simulink model "SF014A_InertiaCmpVel"  (R2013b)
settings: Solver=FixedStepDiscrete  SolverMode=SingleTasking  StartTime=0.0  StopTime=10  FixedStep=0.002  RelTol=1e-3
undefined symbols (not defined in the file): ARCHGLBPRM_2MILLISEC_SEC_F32, ARCHGLBPRM_2PI_ULS_F32, ARCHGLBPRM_PIOVER180_ULS_F32, FLTINJ_INERTIACMPVEL_INERTIACMPCMD, InertiaCmpVelDampgDecelGain, InertiaCmpVelDampgDecelGainFallSlew, InertiaCmpVelDampgGainOffThd, InertiaCmpVelDampgGainOnThd, InertiaCmpVelDecelGainEnaCal, InertiaCmpVelMotInertia, InertiaCmpVelNotchFilStruct, NOTCHFILZEROTHD_ULS_F32, SysGlbPrmSysKineRat, SysGlbPrmTorsBarStfn
libraries: FixdToFloat x13, LnrIntrpn x13, FloatToFixd x9, NxtrAbslt x4, NxtrMath x4, NxtrLim x4, simulink x2, Fil x2
(part 1 of 3)
Description:
  | Provide compensation that is dependent on filtering of motor velocity.  Primary purpose is to compensate for motor inertia
  | at low frequencies and provide damping acting at higher frequencies.
  | 
  | This function requires SF-00 Common Calibrations.
settings Model: Creator=xzqqlw  LastModifiedBy=XZB1DB
settings SolverCC: AutoInsertRateTranBlk=on  InsertRTBMode=Always
settings DataIOCC: LimitDataPoints=off  SaveFormat=Structure  ReturnWorkspaceOutputs=on
settings OptimizationCC: BlockReduction=off  InlineParams=on  ZeroExternalMemoryAtStartup=off  ZeroInternalMemoryAtStartup=off  OptimizeModelRefInitCode=on  LifeSpan=1
settings DebuggingCC: SignalInfNanChecking=error  SignalRangeChecking=warning  UnderspecifiedInitializationDetection=Simplified  SolverPrmCheckMsg=error  InheritedTsInSrcMsg=error  DiscreteInheritContinuousMsg=error  SingleTaskRateTransMsg=error  TasksWithSamePriorityMsg=error  SigSpecEnsureSampleTimeMsg=error  CheckMatrixSingularityMsg=error  ParameterUnderflowMsg=error  ParameterPrecisionLossMsg=error  ParameterTunabilityLossMsg=error  FixptConstUnderflowMsg=warning  FixptConstOverflowMsg=warning  VectorMatrixConversionMsg=error  SignalLabelMismatchMsg=error  UnconnectedInputMsg=error  UnconnectedOutputMsg=error  UnconnectedLineMsg=error  SFcnCompatibilityMsg=error  UniqueDataStoreMsg=warning  BusObjectLabelMismatch=error  RootOutportRequireBusObject=error  AssertControl=DisableAll  ModelReferenceIOMsg=error  ModelReferenceVersionMismatchMessage=warning  ModelReferenceIOMismatchMessage=error  ModelReferenceCSMismatchMessage=warning  ModelReferenceDataLoggingMessage=error  StateNameClashWarn=warning  StrictBusMsg=ErrorOnBusTreatedAsVector  NonBusSignalsTreatedAsBus=error  SFUnexpectedBacktrackingDiag=error  SFInvalidInputDataAccessInChartInitDiag=error  SFNoUnconditionalDefaultTransitionDiag=error  SFTransitionOutsideNaturalParentDiag=error  SFUnconditionalTransitionShadowingDiag=error  SFUndirectedBroadcastEventsDiag=error
settings ModelReferenceCC: ModelReferenceNumInstancesAllowed=Single
settings RTWCC: SystemTargetFile=autosar.tlc  GenCodeOnly=on  TemplateMakefile=ert_default_tmf  Description=AUTOSAR  GenerateReport=on  ProcessScript=autosar_make_rtw_hook  LaunchReport=on
settings CodeAppCC: GenerateComments=off  IgnoreCustomStorageClasses=off  CustomSymbolStrType=$N$R$M  CustomSymbolStrBlkIO=$N$M  SimulinkBlockComments=off
settings STFCustomTargetCC: ParMdlRefBuildCompliant=on  CompOptLevelCompliant=on  IncludeMdlTerminateFcn=off  CombineOutputUpdateFcns=on  SuppressErrorStatus=on  ERTFirstTimeCompliant=on  ERTCustomFileBanners=on  SupportNonFinite=off  SupportComplex=off  SupportContinuousTime=off  SupportNonInlinedSFcns=off  MATLABClassNameForMDSCustomization=Simulink.SoftwareTarget.ERTCustomization  AutosarCompliant=on  GRTInterface=off  SystemTargetFile=autosar.tlc
settings ERTTargetCC: CodeReplacementLibrary=ANSI_C  ConcurrentExecutionCompliant=off  IncludeMdlTerminateFcn=off  SuppressErrorStatus=on  SupportNonFinite=off  SupportComplex=off  ModelStepFunctionPrototypeControlCompliant=off  CPPClassGenCompliant=off  AutosarCompliant=on  InlinedParameterPlacement=NonHierarchical  ERTCustomFileTemplate=example_file_process.tlc  EnableUserReplacementTypes=on

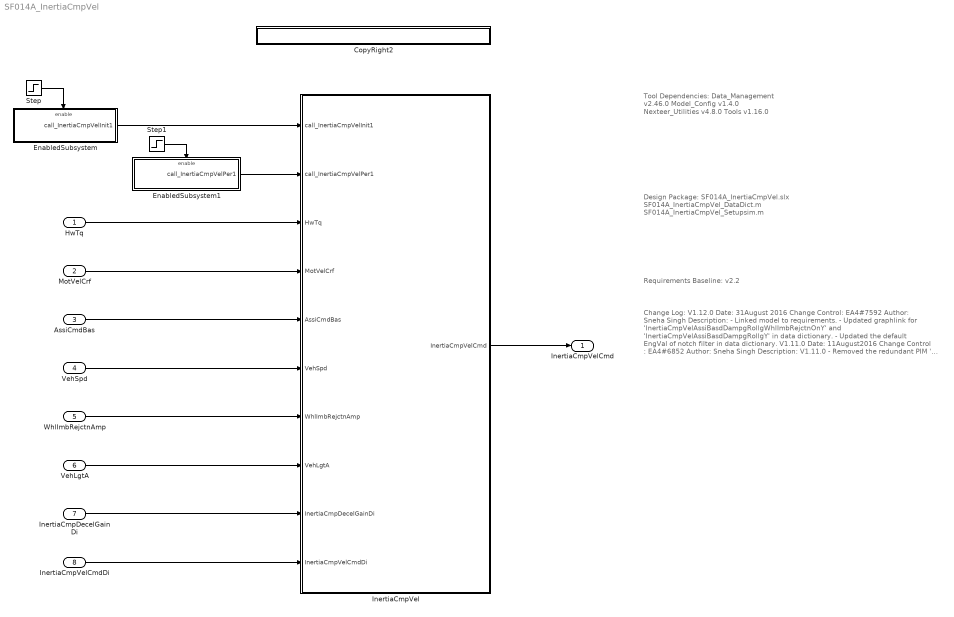
== system SF014A_InertiaCmpVel ==
  note: Requirements Baseline: v2.2
  note: Design Package:
      | SF014A_InertiaCmpVel.slx
      | SF014A_InertiaCmpVel_DataDict.m
      | SF014A_InertiaCmpVel_Setupsim.m
  note: Tool Dependencies:
      |
      | Data_Management v2.46.0
      | Model_Config v1.4.0
      | Nexteer_Utilities v4.8.0
      | Tools v1.16.0
  note: Change Log:
      |
      | V1.12.0
      | Date: 31August 2016
      | Change Control: EA4#7592
      | Author: Sneha Singh
      | Description:
      | - Linked model to requirements.
      | - Updated graphlink for 'InertiaCmpVelAssiBasdDampgRollgWhlImbRejctnOnY' and
      | 'InertiaCmpVelAssiBasdDampgRollgY' in data dictionary.
      | - Updated the default EngVal of notch filter in data dictionary.
      |
      | V1.11.0
      | Date: 11August2016
      | Change Control : EA4#6852
      | Author: Sneha Singh
      |
      | Description:
      | V1.11.0
      | - Removed the redundant PIM ' DecelGainPrev' and the display variable 'dInertiaCmpVelDecelGain '.
      | V1.10.0
      | - Conversion from Level 0 to Level 3 model.
      | - Names of PIM blocks have been updated as per EA4 standards in model and DD.
      | - Range of Filter Gain and State Variable for 'TqSnsrVelFil' updated in the data dictionary.
      | - Added the graphlink property for 'InertiaCmpVelNotchBlndY' in the data dictionary.
      | V1.9.0
      | - Modified datatype of Input 'InertiaCmpDecelGainDi' in the data dictionary.
      | - Added the Cal 'InertiaCmpVelDecelGainEnaCal' to data dictionary and model.
      | V1.8.0
      | - Modified datatype of PIM variable 'NotchFilChk'
      | V1.7.0
      | - Added the PIM variable 'NotchFilChk'
      | - Modified the 'Inertia Comp Notch Compensation' block.
      | - Added a saturation block to the velocity output in the block 'DriverVelCalc'.
      | Added a saturation block to the Inertia Comp output in the block 'GenFddIcCmd'.
      | - Added the input 'InertiaCmpDecelGainDi' to the model.
      | - Changes in the limits of some PIM variables in data dictionary.
      | V1.6.0
      | - Few simulink model properties changed (specifically initial conditions)
      |  so that the simulation can run.
      | - Changes in the limits of some PIM variables in data dictionary.
      | V1.5.0
      | - DriverVelCalc block modified to add motor velocity for the output (Simulink
      | model/design modification)
      | - Changes in the limits of some PIM variables in data dictionary.
      | - The min/max and default value of InertiaCmpVelDampgDecelGainFallSlew
      | V1.4.0
      | - Changes in the limits of some display variables in data dictionary.
      | - Few simulink model properties changes so that the simulation can run.
      | V1.3.0
      | - No changes to model or data dictionary.
      | - Added an init.txt file for initialization
      | were modified in data dictionary.
      | V1.2.0
      | - Minor changes to data dictionary
      |  and default cals.
      | V1.1.0
      | - Minor changes to data dictionary
      | V1.0.0
      | - Initial Release
      | - Based on EA3 version 006
      | - Notch Filter Added
  HwTq : Inport  OutDataTypeStr=single
  MotVelCrf : Inport  Port=2  OutDataTypeStr=single
  AssiCmdBas : Inport  Port=3  OutDataTypeStr=single
  VehSpd : Inport  Port=4  OutDataTypeStr=single
  WhlImbRejctnAmp : Inport  Port=5  OutDataTypeStr=single
  VehLgtA : Inport  Port=6  OutDataTypeStr=single
  InertiaCmpDecelGainDi : Inport  Port=7  OutDataTypeStr=single
  InertiaCmpVelCmdDi : Inport  Port=8  OutDataTypeStr=single
  CopyRight2 : Subsystem  Description=|  mask(Copyright Information){none=on}
      | Copyright info block.                                               
      |                                                                     
      | Place copyright information at the top of every subsystem in design.
      mask prompts: none "No parameters"
      mask help: Place copyright information at the top of every subsystem in design.
      mask Display:
      | NxtrConf = 'Nexteer Confidential';
      | 
      | sys = bdroot; %handle for the current model ("system")
      | first = get_param(sys,'Created');
      | first = first(end-3:end);  %year is last four digits
      | 
      | last = get_param(sys,'LastModifiedDate');
      | if isempty(last)
      |     last = datestr(now,'yyyy');
      | else
      |     last = last(end-3:end);
      | end
      | 
      | if strcmp(first,last)
      |     fprintf('%s -- Copyright %s Nexteer',NxtrConf,first)
      | else
      |     fprintf('%s -- %s%s- %s Nexteer',NxtrConf,char(169),first,last)
      | end
  EnabledSubsystem : Subsystem  TreatAsAtomicUnit=on
  EnabledSubsystem1 : Subsystem  TreatAsAtomicUnit=on
  InertiaCmpVel : Subsystem
  Step : Step  Time=0  Before=1  After=0  SampleTime=0
  Step1 : Step  Time=0  SampleTime=0.002
  InertiaCmpVelCmd : Outport
  wires:
  AssiCmdBas/1 -> InertiaCmpVel/5(AssiCmdBas)
  VehSpd/1 -> InertiaCmpVel/6(VehSpd)
  WhlImbRejctnAmp/1 -> InertiaCmpVel/7(WhlImbRejctnAmp)
  HwTq/1 -> InertiaCmpVel/3(HwTq)
  MotVelCrf/1 -> InertiaCmpVel/4(MotVelCrf)
  InertiaCmpVel/1(InertiaCmpVelCmd) -> InertiaCmpVelCmd/1
  InertiaCmpVelCmdDi/1 -> InertiaCmpVel/10(InertiaCmpVelCmdDi)
  VehLgtA/1 -> InertiaCmpVel/8(VehLgtA)
  Step/1 -> EnabledSubsystem/Enable
  EnabledSubsystem1/1(call_InertiaCmpVelPer1) -> InertiaCmpVel/2(call_InertiaCmpVelPer1)
  EnabledSubsystem/1(call_InertiaCmpVelInit1) -> InertiaCmpVel/1(call_InertiaCmpVelInit1)
  Step1/1 -> EnabledSubsystem1/Enable
  InertiaCmpDecelGainDi/1 -> InertiaCmpVel/9(InertiaCmpDecelGainDi)

== system SF014A_InertiaCmpVel/CopyRight2 ==

== system SF014A_InertiaCmpVel/EnabledSubsystem ==
  Enable : EnablePort
  CopyRight2 : Subsystem  Description=|  mask(Copyright Information){none=on}
      | Copyright info block.                                               
      |                                                                     
      | Place copyright information at the top of every subsystem in design.
      mask prompts: none "No parameters"
      mask help: Place copyright information at the top of every subsystem in design.
      mask Display:
      | NxtrConf = 'Nexteer Confidential';
      | 
      | sys = bdroot; %handle for the current model ("system")
      | first = get_param(sys,'Created');
      | if(isempty(first))
      |     first = datestr(now,'yyyy');
      | else
      |     first = first(end-3:end);  %year is last four digits
      | end
      | 
      | last = get_param(sys,'LastModifiedDate');
      | if isempty(last)
      |     last = datestr(now,'yyyy');
      | else
      |     last = last(end-3:end);
      | end
      | 
      | if strcmp(first,last)
      |     fprintf('%s -- Copyright %s Nexteer',NxtrConf,first)
      | else
      |     fprintf('%s -- %s%s- %s Nexteer',NxtrConf,char(169),first,last)
      | end
  Function-Call Generator1 : simulink/Ports & Subsystems/Function-Call Generator  sample_time=0  numberOfIterations=1
  call_InertiaCmpVelInit1 : Outport
  wires:
  Function-Call Generator1/1 -> call_InertiaCmpVelInit1/1

== system SF014A_InertiaCmpVel/EnabledSubsystem1 ==
  Enable : EnablePort
  CopyRight2 : Subsystem  Description=|  mask(Copyright Information){none=on}
      | Copyright info block.                                               
      |                                                                     
      | Place copyright information at the top of every subsystem in design.
      mask prompts: none "No parameters"
      mask help: Place copyright information at the top of every subsystem in design.
      mask Display:
      | NxtrConf = 'Nexteer Confidential';
      | 
      | sys = bdroot; %handle for the current model ("system")
      | first = get_param(sys,'Created');
      | if(isempty(first))
      |     first = datestr(now,'yyyy');
      | else
      |     first = first(end-3:end);  %year is last four digits
      | end
      | 
      | last = get_param(sys,'LastModifiedDate');
      | if isempty(last)
      |     last = datestr(now,'yyyy');
      | else
      |     last = last(end-3:end);
      | end
      | 
      | if strcmp(first,last)
      |     fprintf('%s -- Copyright %s Nexteer',NxtrConf,first)
      | else
      |     fprintf('%s -- %s%s- %s Nexteer',NxtrConf,char(169),first,last)
      | end
  Function-Call Generator1 : simulink/Ports & Subsystems/Function-Call Generator  sample_time=0.002  numberOfIterations=1
  call_InertiaCmpVelPer1 : Outport
  wires:
  Function-Call Generator1/1 -> call_InertiaCmpVelPer1/1

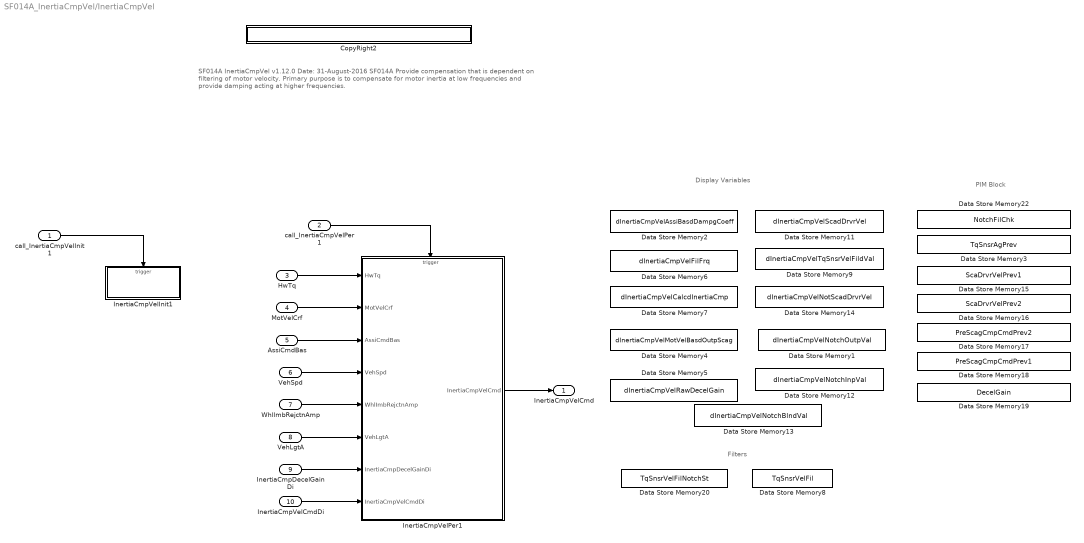
== system SF014A_InertiaCmpVel/InertiaCmpVel ==
  note: Display Variables
  note: SF014A  InertiaCmpVel
      | v1.12.0 														Date: 31-August-2016
      |
      | SF014A
      | Provide compensation that is dependent on filtering
      | of motor velocity. Primary purpose is to compensate for motor inertia at
      | low frequencies and provide damping acting at higher frequencies.
  note: PIM Block
  note: Filters
  call_InertiaCmpVelInit1 : Inport
  call_InertiaCmpVelPer1 : Inport  Port=2
  HwTq : Inport  RequirementInfo="{'linktype_rmi_doors' '0000a52e (/E-STEER Core/SubSystem Specifications/Application Functions/SF014A Inertia Compensation)' '#SF014A_9' 'true' 'REQ:  SF014A_9' '' } %GIDa_f01b9146_b334_492a_9ec3_b1b2beaf36fa"  Port=3  OutDataTypeStr=single
  MotVelCrf : Inport  RequirementInfo="{'linktype_rmi_doors' '0000a52e (/E-STEER Core/SubSystem Specifications/Application Functions/SF014A Inertia Compensation)' '#SF014A_32' 'true' 'REQ:  SF014A_32' '' } %GIDa_a3fb682f_8b72_444f_8c20_ec5397ad6a39"  Port=4  OutDataTypeStr=single
  AssiCmdBas : Inport  RequirementInfo="{'linktype_rmi_doors' '0000a52e (/E-STEER Core/SubSystem Specifications/Application Functions/SF014A Inertia Compensation)' '#SF014A_33' 'true' 'REQ:  SF014A_33' '' } %GIDa_d5627f17_e36b_4ebf_b0c3_bf571987fd69"  Port=5  OutDataTypeStr=single
  VehSpd : Inport  RequirementInfo="{'linktype_rmi_doors' '0000a52e (/E-STEER Core/SubSystem Specifications/Application Functions/SF014A Inertia Compensation)' '#SF014A_34' 'true' 'REQ:  SF014A_34' '' } %GIDa_30fe50f3_e3d5_4c85_a02f_97c34158807d"  Port=6  OutDataTypeStr=single
  WhlImbRejctnAmp : Inport  RequirementInfo="{'linktype_rmi_doors' '0000a52e (/E-STEER Core/SubSystem Specifications/Application Functions/SF014A Inertia Compensation)' '#SF014A_35' 'true' 'REQ:  SF014A_35' '' } %GIDa_6689df3e_a07a_4416_91b0_faa74f28addd"  Port=7  OutDataTypeStr=single
  VehLgtA : Inport  RequirementInfo="{'linktype_rmi_doors' '0000a52e (/E-STEER Core/SubSystem Specifications/Application Functions/SF014A Inertia Compensation)' '#SF014A_37' 'true' 'REQ:  SF014A_37' '' } %GIDa_068774d9_b29a_42bf_9303_5199fc3935e8"  Port=8  OutDataTypeStr=single
  InertiaCmpDecelGainDi : Inport  RequirementInfo="{'linktype_rmi_doors' '0000a52e (/E-STEER Core/SubSystem Specifications/Application Functions/SF014A Inertia Compensation)' '#SF014A_64' 'true' 'REQ:  SF014A_64' '' } %GIDa_847a8fc7_5162_4283_91ca_d0e4dd3290d5"  Port=9  OutDataTypeStr=single
  InertiaCmpVelCmdDi : Inport  RequirementInfo="{'linktype_rmi_doors' '0000a52e (/E-STEER Core/SubSystem Specifications/Application Functions/SF014A Inertia Compensation)' '#SF014A_36' 'true' 'REQ:  SF014A_36' '' } %GIDa_8753a04c_012b_41bc_9ba5_be465b9c35dc"  Port=10  OutDataTypeStr=single
  CopyRight2 : Subsystem  Description=|  mask(Copyright Information){none=on}
      | Copyright info block.                                               
      |                                                                     
      | Place copyright information at the top of every subsystem in design.
      mask prompts: none "No parameters"
      mask help: Place copyright information at the top of every subsystem in design.
      mask Display:
      | NxtrConf = 'Nexteer Confidential';
      | 
      | sys = bdroot; %handle for the current model ("system")
      | first = get_param(sys,'Created');
      | first = first(end-3:end);  %year is last four digits
      | 
      | last = get_param(sys,'LastModifiedDate');
      | if isempty(last)
      |     last = datestr(now,'yyyy');
      | else
      |     last = last(end-3:end);
      | end
      | 
      | if strcmp(first,last)
      |     fprintf('%s -- Copyright %s Nexteer',NxtrConf,first)
      | else
      |     fprintf('%s -- %s%s- %s Nexteer',NxtrConf,char(169),first,last)
      | end
  Data Store Memory1 : DataStoreMemory  DataStoreName=dInertiaCmpVelNotchOutpVal  ReadBeforeWriteMsg=warning  WriteAfterWriteMsg=warning  WriteAfterReadMsg=warning  StateMustResolveToSignalObject=on
  Data Store Memory11 : DataStoreMemory  DataStoreName=dInertiaCmpVelScadDrvrVel  ReadBeforeWriteMsg=warning  WriteAfterWriteMsg=warning  WriteAfterReadMsg=warning  StateMustResolveToSignalObject=on
  Data Store Memory12 : DataStoreMemory  DataStoreName=dInertiaCmpVelNotchInpVal  ReadBeforeWriteMsg=warning  WriteAfterWriteMsg=warning  WriteAfterReadMsg=warning  StateMustResolveToSignalObject=on
  Data Store Memory13 : DataStoreMemory  DataStoreName=dInertiaCmpVelNotchBlndVal  ReadBeforeWriteMsg=warning  WriteAfterWriteMsg=warning  WriteAfterReadMsg=warning  StateMustResolveToSignalObject=on
  Data Store Memory14 : DataStoreMemory  DataStoreName=dInertiaCmpVelNotScadDrvrVel  ReadBeforeWriteMsg=warning  WriteAfterWriteMsg=warning  WriteAfterReadMsg=warning  StateMustResolveToSignalObject=on
  Data Store Memory15 : DataStoreMemory  DataStoreName=ScaDrvrVelPrev1  StateMustResolveToSignalObject=on
  Data Store Memory16 : DataStoreMemory  DataStoreName=ScaDrvrVelPrev2  StateMustResolveToSignalObject=on
  Data Store Memory17 : DataStoreMemory  DataStoreName=PreScagCmpCmdPrev2  StateMustResolveToSignalObject=on
  Data Store Memory18 : DataStoreMemory  DataStoreName=PreScagCmpCmdPrev1  StateMustResolveToSignalObject=on
  Data Store Memory19 : DataStoreMemory  DataStoreName=DecelGain  StateMustResolveToSignalObject=on
  Data Store Memory2 : DataStoreMemory  DataStoreName=dInertiaCmpVelAssiBasdDampgCoeff  ReadBeforeWriteMsg=warning  WriteAfterWriteMsg=warning  WriteAfterReadMsg=warning  StateMustResolveToSignalObject=on
  Data Store Memory20 : DataStoreMemory  DataStoreName=TqSnsrVelFilNotchSt  ReadBeforeWriteMsg=warning  WriteAfterWriteMsg=warning  WriteAfterReadMsg=warning  InitialValue=[]  StateMustResolveToSignalObject=on
  Data Store Memory22 : DataStoreMemory  RequirementInfo="{'linktype_rmi_doors' '0000a52e (/E-STEER Core/SubSystem Specifications/Application Functions/SF014A Inertia Compensation)' '#SF014A_94' 'true' 'REQ:  SF014A_94' '' } %GIDa_2f01161b_bb81_48fb_9c8e_b5cf915a9566"  DataStoreName=NotchFilChk  StateMustResolveToSignalObject=on
  Data Store Memory3 : DataStoreMemory  DataStoreName=TqSnsrAgPrev  StateMustResolveToSignalObject=on
  Data Store Memory4 : DataStoreMemory  DataStoreName=dInertiaCmpVelMotVelBasdOutpScag  ReadBeforeWriteMsg=warning  WriteAfterWriteMsg=warning  WriteAfterReadMsg=warning  StateMustResolveToSignalObject=on
  Data Store Memory5 : DataStoreMemory  DataStoreName=dInertiaCmpVelRawDecelGain  ReadBeforeWriteMsg=warning  WriteAfterWriteMsg=warning  WriteAfterReadMsg=warning  StateMustResolveToSignalObject=on
  Data Store Memory6 : DataStoreMemory  DataStoreName=dInertiaCmpVelFilFrq  ReadBeforeWriteMsg=warning  WriteAfterWriteMsg=warning  WriteAfterReadMsg=warning  StateMustResolveToSignalObject=on
  Data Store Memory7 : DataStoreMemory  DataStoreName=dInertiaCmpVelCalcdInertiaCmp  ReadBeforeWriteMsg=warning  WriteAfterWriteMsg=warning  WriteAfterReadMsg=warning  StateMustResolveToSignalObject=on
  Data Store Memory8 : DataStoreMemory  DataStoreName=TqSnsrVelFil  InitialValue=[]  OutDataTypeStr=Bus: FilLpRec1  StateMustResolveToSignalObject=on
  Data Store Memory9 : DataStoreMemory  DataStoreName=dInertiaCmpVelTqSnsrVelFildVal  ReadBeforeWriteMsg=warning  WriteAfterWriteMsg=warning  WriteAfterReadMsg=warning  StateMustResolveToSignalObject=on
  InertiaCmpVelInit1 : Subsystem  TreatAsAtomicUnit=on
  InertiaCmpVelPer1 : Subsystem
  InertiaCmpVelCmd : Outport  RequirementInfo="{'linktype_rmi_doors' '0000a52e (/E-STEER Core/SubSystem Specifications/Application Functions/SF014A Inertia Compensation)' '#SF014A_11' 'true' 'REQ:  SF014A_11' '' } %GIDa_b766a6be_ddbc_4ccc_baa7_69f83a871e7a"
  wires:
  InertiaCmpVelPer1/1(InertiaCmpVelCmd) -> InertiaCmpVelCmd/1
  AssiCmdBas/1 -> InertiaCmpVelPer1/3(AssiCmdBas)
  VehSpd/1 -> InertiaCmpVelPer1/4(VehSpd)
  VehLgtA/1 -> InertiaCmpVelPer1/6(VehLgtA)
  InertiaCmpVelCmdDi/1 -> InertiaCmpVelPer1/8(InertiaCmpVelCmdDi)
  WhlImbRejctnAmp/1 -> InertiaCmpVelPer1/5(WhlImbRejctnAmp)
  HwTq/1 -> InertiaCmpVelPer1/1(HwTq)
  MotVelCrf/1 -> InertiaCmpVelPer1/2(MotVelCrf)
  call_InertiaCmpVelInit1/1 -> InertiaCmpVelInit1/Trigger
  call_InertiaCmpVelPer1/1 -> InertiaCmpVelPer1/Trigger
  InertiaCmpDecelGainDi/1 -> InertiaCmpVelPer1/7(InertiaCmpDecelGainDi)

== system SF014A_InertiaCmpVel/EnabledSubsystem/CopyRight2 ==

== system SF014A_InertiaCmpVel/EnabledSubsystem1/CopyRight2 ==

== system SF014A_InertiaCmpVel/InertiaCmpVel/CopyRight2 ==

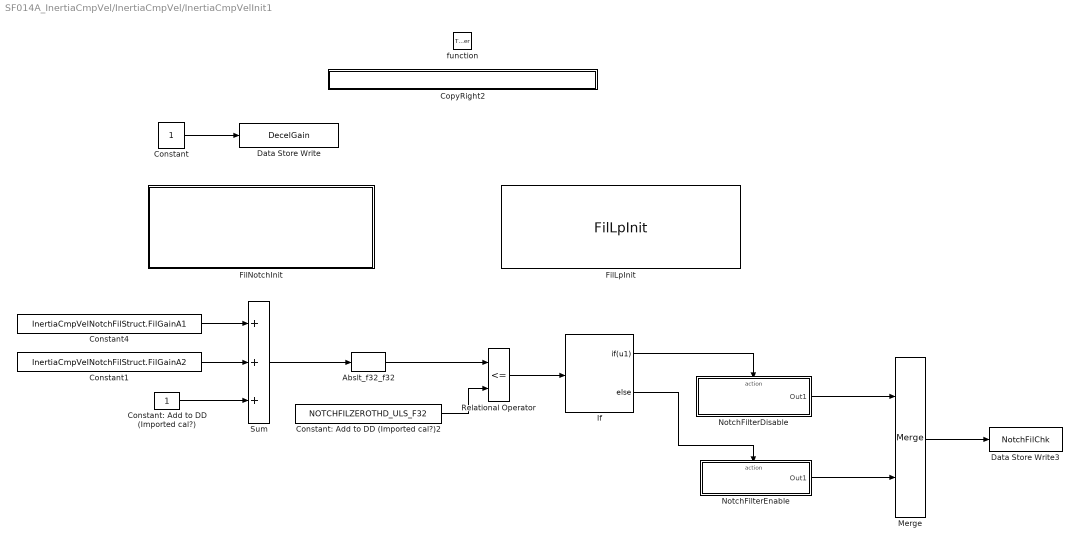
== system SF014A_InertiaCmpVel/InertiaCmpVel/InertiaCmpVelInit1 ==
  function : TriggerPort  TriggerType=function-call
  Abslt_f32_f32 : NxtrAbslt/Abslt_f32_f32  RequirementInfo="{'linktype_rmi_doors' '0000a52e (/E-STEER Core/SubSystem Specifications/Application Functions/SF014A Inertia Compensation)' '#SF014A_95' 'true' 'REQ:  SF014A_95' '' } %GIDa_2b983676_40f4_4fb6_a890_543181c91400"  SFunctionSpec=single y1 = Abslt_f32_f32(single u1)
      settings: AttributesFormatString=%<Name>
  Constant : Constant  OutDataTypeStr=single
      settings: AttributesFormatString=%<OutDataTypeStr>
  Constant1 : Constant  RequirementInfo="{'linktype_rmi_doors' '0000a52e (/E-STEER Core/SubSystem Specifications/Application Functions/SF014A Inertia Compensation)' '#SF014A_95' 'true' 'REQ:  SF014A_95' '' } %GIDa_ae310083_699d_4c0c_9a75_6c389a9a4f0b"  Value=InertiaCmpVelNotchFilStruct.FilGainA2
  Constant4 : Constant  RequirementInfo="{'linktype_rmi_doors' '0000a52e (/E-STEER Core/SubSystem Specifications/Application Functions/SF014A Inertia Compensation)' '#SF014A_95' 'true' 'REQ:  SF014A_95' '' } %GIDa_4f0e092c_5676_4daa_912b_2ece80eb9d0f"  Value=InertiaCmpVelNotchFilStruct.FilGainA1
  Constant: Add to DD (Imported cal?) : Constant  RequirementInfo="{'linktype_rmi_doors' '0000a52e (/E-STEER Core/SubSystem Specifications/Application Functions/SF014A Inertia Compensation)' '#SF014A_95' 'true' 'REQ:  SF014A_95' '' } %GIDa_21caba87_9a90_4748_8ac1_f3e85f9c4cfc"  OutDataTypeStr=single
      settings: AttributesFormatString=%<OutDataTypeStr>
  Constant: Add to DD (Imported cal?)2 : Constant  RequirementInfo="{'linktype_rmi_doors' '0000a52e (/E-STEER Core/SubSystem Specifications/Application Functions/SF014A Inertia Compensation)' '#SF014A_95' 'true' 'REQ:  SF014A_95' '' } %GIDa_b08a34eb_afdb_4d33_b51b_58cf003e6c96"  Value=NOTCHFILZEROTHD_ULS_F32  OutDataTypeStr=double
  CopyRight2 : Subsystem  Description=|  mask(Copyright Information){none=on}
      | Copyright info block.                                               
      |                                                                     
      | Place copyright information at the top of every subsystem in design.
      mask prompts: none "No parameters"
      mask help: Place copyright information at the top of every subsystem in design.
      mask Display:
      | NxtrConf = 'Nexteer Confidential';
      | 
      | sys = bdroot; %handle for the current model ("system")
      | first = get_param(sys,'Created');
      | first = first(end-3:end);  %year is last four digits
      | 
      | last = get_param(sys,'LastModifiedDate');
      | if isempty(last)
      |     last = datestr(now,'yyyy');
      | else
      |     last = last(end-3:end);
      | end
      | 
      | if strcmp(first,last)
      |     fprintf('%s -- Copyright %s Nexteer',NxtrConf,first)
      | else
      |     fprintf('%s -- %s%s- %s Nexteer',NxtrConf,char(169),first,last)
      | end
  Data Store Write : DataStoreWrite  DataStoreName=DecelGain
  Data Store Write3 : DataStoreWrite  RequirementInfo="{'linktype_rmi_doors' '0000a52e (/E-STEER Core/SubSystem Specifications/Application Functions/SF014A Inertia Compensation)' '#SF014A_95' 'true' 'REQ:  SF014A_95' '' } %GIDa_18677b43_f415_4657_9de0_d1455a2ff15d"  DataStoreName=NotchFilChk
  FilLpInit : Fil/FilLpInit  Ic=0  Ts=ARCHGLBPRM_2MILLISEC_SEC_F32  Freq=InertiaCmpVelTqSnsrVelFilFrq  StVar=TqSnsrVelFil
  FilNotchInit : Subsystem  mask(FilNotchInit){StVarGain=InertiaCmpVelNotchFilStruct, StVarSt=TqSnsrVelFilNotchSt}
      mask prompts: StVarGain "State Variable For Gain"; StVarSt "State Variable For State"
      mask help: It Initializes filter states
      mask init:
      | blk = gcb;
      | set_param([ blk '/Constant2'],'Value',[StVarGain '.FilGainB1'])
      | set_param([ blk '/Constant3'],'Value',[StVarGain '.FilGainB2'])
      | set_param([ blk '/Constant4'],'Value',[StVarGain '.FilGainA1'])
      | set_param([ blk '/Constant5'],'Value',[StVarGain '.FilGainA2'])
      | set_param([ blk '/Constant6'],'Value',[StVarGain '.FilGainB2'])
      | set_param([ blk '/Constant7'],'Value',[StVarGain '.FilGainA2'])
      | set_param([ blk '/Data Store Write'],'DataStoreName',StVarSt)
      | set_param([ blk '/Data Store Write1'],'DataStoreName',StVarSt)
      | 
      | try
      |     dt = evalin('base',[StVarGain '.EngDT']);
      | catch err
      |     if strcmp(err.identifier,'MATLAB:undefinedVarOrClass')
      |         dt = struct.FilNotchGainRec1;
      |     end
      | end
      | 
      | try
      |     dt1 = evalin('base',[StVarSt '.EngDT']);
      | catch err
      |     if strcmp(err.identifier,'MATLAB:undefinedVarOrClass')
      |         dt1 = struct.FilNotchStRec1;
      |     end
      | end
      | 
      | 
      | if isa(dt1,'struct.FilNotchStRec1')
      |     set_param([ blk '/Data Store Write'],'DataStoreElements',[StVarSt '.FilSt1'])
      |     set_param([ blk '/Data Store Write1'],'DataStoreElements',[StVarSt '.FilSt2'])
      |     
      | else
      |     error('Incorrect data class.');
      | end
      settings: AttributesFormatString=%<Tag>
      mask Display:
      | text(0.35,0.9,'FilNotchInit')
      | text(0.05,0.5,['StVarForGain: ' StVarGain])
      | text(0.05,0.2,['StVarForSt: ' StVarSt])
  If : If  RequirementInfo="{'linktype_rmi_doors' '0000a52e (/E-STEER Core/SubSystem Specifications/Application Functions/SF014A Inertia Compensation)' '#SF014A_95' 'true' 'REQ:  SF014A_95' '' } %GIDa_b9cdf93b_f7a8_4fa6_8e24_79d43f4b5c6d"  IfExpression=u1
  Merge : Merge  RequirementInfo="{'linktype_rmi_doors' '0000a52e (/E-STEER Core/SubSystem Specifications/Application Functions/SF014A Inertia Compensation)' '#SF014A_95' 'true' 'REQ:  SF014A_95' '' } %GIDa_6b42e7b3_58c6_47fa_88af_57c14584b984"
  NotchFilterDisable : Subsystem  RequirementInfo="{'linktype_rmi_doors' '0000a52e (/E-STEER Core/SubSystem Specifications/Application Functions/SF014A Inertia Compensation)' '#SF014A_95' 'true' 'REQ:  SF014A_95' '' } %GIDa_c8bf08d4_750c_417c_aa6d_701d4f336508"  TreatAsAtomicUnit=on
  NotchFilterEnable : Subsystem  TreatAsAtomicUnit=on
  Relational Operator : RelationalOperator  RequirementInfo="{'linktype_rmi_doors' '0000a52e (/E-STEER Core/SubSystem Specifications/Application Functions/SF014A Inertia Compensation)' '#SF014A_95' 'true' 'REQ:  SF014A_95' '' } %GIDa_c3b30c81_22ab_481d_a60b_2436f534e91d"  Operator=<=  OutDataTypeStr=boolean
  Sum : Sum  RequirementInfo="{'linktype_rmi_doors' '0000a52e (/E-STEER Core/SubSystem Specifications/Application Functions/SF014A Inertia Compensation)' '#SF014A_95' 'true' 'REQ:  SF014A_95' '' } %GIDa_3f306fac_caeb_431d_a817_48d914465659"  Inputs=+++
  wires:
  Constant/1 -> Data Store Write/1
  Constant: Add to DD (Imported cal?)/1 -> Sum/3
  Constant1/1 -> Sum/2
  Constant4/1 -> Sum/1
  Sum/1 -> Abslt_f32_f32/1
  Merge/1 -> Data Store Write3/1
  NotchFilterDisable/1(Out1) -> Merge/1
  NotchFilterEnable/1(Out1) -> Merge/2
  Relational Operator/1 -> If/1
  Abslt_f32_f32/1 -> Relational Operator/1
  Constant: Add to DD (Imported cal?)2/1 -> Relational Operator/2
  If/1 -> NotchFilterDisable/Action
  If/2 -> NotchFilterEnable/Action

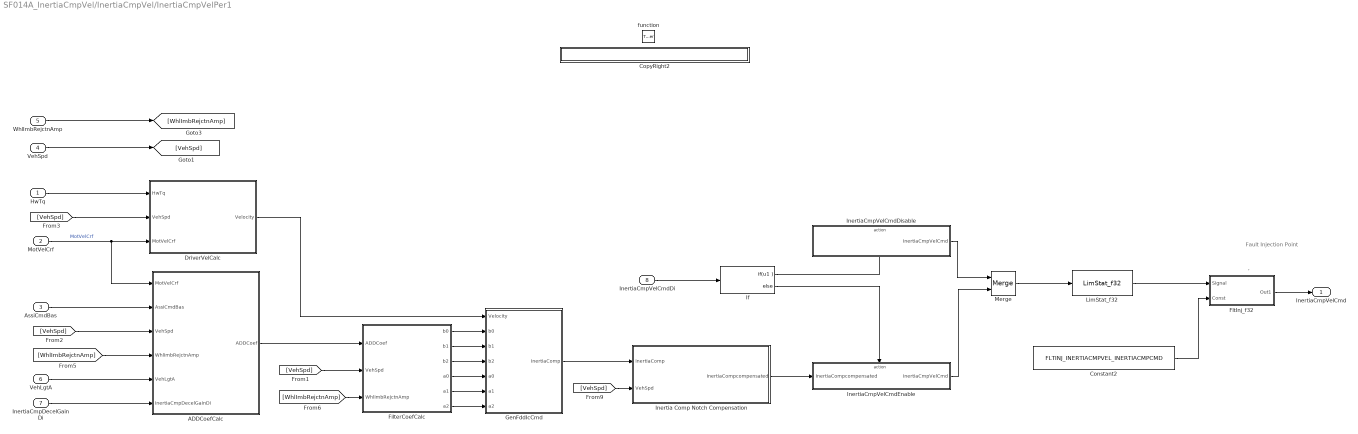
== system SF014A_InertiaCmpVel/InertiaCmpVel/InertiaCmpVelPer1 ==
  note: ,
  note: Fault
      | Injection
      | Point
  HwTq : Inport
  MotVelCrf : Inport  Port=2
  AssiCmdBas : Inport  Port=3
  VehSpd : Inport  Port=4
  WhlImbRejctnAmp : Inport  Port=5
  VehLgtA : Inport  Port=6
  InertiaCmpDecelGainDi : Inport  Port=7
  InertiaCmpVelCmdDi : Inport  RequirementInfo="{'linktype_rmi_doors' '0000a52e (/E-STEER Core/SubSystem Specifications/Application Functions/SF014A Inertia Compensation)' '#SF014A_61' 'true' 'REQ:  SF014A_61' '' } %GIDa_0bbec89a_36ee_4b95_b953_11359f7044df"  Port=8
  function : TriggerPort  TriggerType=function-call
  ADDCoefCalc : Subsystem  Tag=Calculate Assist-Dependent Damping Coefficients  TreatAsAtomicUnit=on
      settings: AttributesFormatString=%<Tag>
  Constant2 : Constant  Value=FLTINJ_INERTIACMPVEL_INERTIACMPCMD
  CopyRight2 : Subsystem  Description=|  mask(Copyright Information){none=on}
      | Copyright info block.                                               
      |                                                                     
      | Place copyright information at the top of every subsystem in design.
      mask prompts: none "No parameters"
      mask help: Place copyright information at the top of every subsystem in design.
      mask Display:
      | NxtrConf = 'Nexteer Confidential';
      | 
      | sys = bdroot; %handle for the current model ("system")
      | first = get_param(sys,'Created');
      | first = first(end-3:end);  %year is last four digits
      | 
      | last = get_param(sys,'LastModifiedDate');
      | if isempty(last)
      |     last = datestr(now,'yyyy');
      | else
      |     last = last(end-3:end);
      | end
      | 
      | if strcmp(first,last)
      |     fprintf('%s -- Copyright %s Nexteer',NxtrConf,first)
      | else
      |     fprintf('%s -- %s%s- %s Nexteer',NxtrConf,char(169),first,last)
      | end
  DriverVelCalc : Subsystem  Tag=Calculate Driver Velocity  Description=Driver Velocity is pinion velocity +/- the effect of T-bar twist.  TreatAsAtomicUnit=on
      settings: AttributesFormatString=%<Tag>
  FilterCoefCalc : Subsystem  Tag=Calculate Filter Coefficients  RequirementInfo="{'linktype_rmi_doors' '0000a52e (/E-STEER Core/SubSystem Specifications/Application Functions/SF014A Inertia Compensation)' '#SF014A_58' 'true' 'REQ:  SF014A_58' '' } %GIDa_a1669d80_7874_4876_b69f_d5b6bd941d92"  TreatAsAtomicUnit=on
      settings: AttributesFormatString=%<Tag>
  FltInj_f32 : Subsystem  RequirementInfo="{'linktype_rmi_doors' '0000a52e (/E-STEER Core/SubSystem Specifications/Application Functions/SF014A Inertia Compensation)' '#SF014A_108' 'true' 'REQ:  SF014A_108' '' } %GIDa_0ede2fb6_9734_4e3a_b1cd_b84e030573e0"  TreatAsAtomicUnit=on  VariantControl=FltInj_sim  mask(Fault_Injection){}
      mask help: Fault Injection is a simulation only block for EA4 programs.
  GenFddIcCmd : Subsystem  Tag=Generate Command  RequirementInfo="{'linktype_rmi_doors' '0000a52e (/E-STEER Core/SubSystem Specifications/Application Functions/SF014A Inertia Compensation)' '#SF014A_83' 'true' 'REQ:  SF014A_83' '' } %GIDa_3d5c9d42_d00c_4853_96e7_696b3e59381c"  TreatAsAtomicUnit=on
      settings: AttributesFormatString=%<Tag>
  If : If  RequirementInfo="{'linktype_rmi_doors' '0000a52e (/E-STEER Core/SubSystem Specifications/Application Functions/SF014A Inertia Compensation)' '#SF014A_61' 'true' 'REQ:  SF014A_61' '' } %GIDa_7de87758_ea01_402d_ab12_9dfc5faf3a8a"  IfExpression=u1
  Inertia Comp Notch Compensation : Subsystem
  InertiaCmpVelCmdDisable : Subsystem  RequirementInfo="{'linktype_rmi_doors' '0000a52e (/E-STEER Core/SubSystem Specifications/Application Functions/SF014A Inertia Compensation)' '#SF014A_61' 'true' 'REQ:  SF014A_61' '' } %GIDa_d2dd46f3_fe51_4fc5_b997_3dceb2949fd3"  TreatAsAtomicUnit=on
  InertiaCmpVelCmdEnable : Subsystem  TreatAsAtomicUnit=on
  LimStat_f32 : NxtrLim/LimStat_f32  RequirementInfo="{'linktype_rmi_doors' '0000a52e (/E-STEER Core/SubSystem Specifications/Application Functions/SF014A Inertia Compensation)' '#SF014A_103' 'true' 'REQ:  SF014A_103' '' } %GIDa_49ff1167_1d1e_4c1b_bde0_f76abb4fb8bf"  LoLim=SYSGLBPRM_MOTTQCMDLOLIM_MOTNWTMTR_F32  HiLim=SYSGLBPRM_MOTTQCMDHILIM_MOTNWTMTR_F32
      settings: AttributesFormatString=|
      | Low Limit: %<LoLim>
      | High Limit:%<HiLim>
  Merge : Merge
  InertiaCmpVelCmd : Outport
  wires:
  FilterCoefCalc/1(b0) -> GenFddIcCmd/2(b0)
  FilterCoefCalc/2(b1) -> GenFddIcCmd/3(b1)
  FilterCoefCalc/3(b2) -> GenFddIcCmd/4(b2)
  FilterCoefCalc/4(a0) -> GenFddIcCmd/5(a0)
  FilterCoefCalc/5(a1) -> GenFddIcCmd/6(a1)
  FilterCoefCalc/6(a2) -> GenFddIcCmd/7(a2)
  ADDCoefCalc/1(ADDCoef) -> FilterCoefCalc/1(ADDCoef)
  [WhlImbRejctnAmp] -> ADDCoefCalc/4(WhlImbRejctnAmp)
  [VehSpd] -> ADDCoefCalc/3(VehSpd)
  MotVelCrf/1 -> ADDCoefCalc/1(MotVelCrf), DriverVelCalc/3(MotVelCrf)  "MotVelCrf"
  DriverVelCalc/1(Velocity) -> GenFddIcCmd/1(Velocity)
  [VehSpd] -> FilterCoefCalc/2(VehSpd)
  [VehSpd] -> DriverVelCalc/2(VehSpd)
  [WhlImbRejctnAmp] -> FilterCoefCalc/3(WhlImbRejctnAmp)
  WhlImbRejctnAmp/1 -> [WhlImbRejctnAmp]
  VehSpd/1 -> [VehSpd]
  HwTq/1 -> DriverVelCalc/1(HwTq)
  AssiCmdBas/1 -> ADDCoefCalc/2(AssiCmdBas)
  VehLgtA/1 -> ADDCoefCalc/5(VehLgtA)
  [VehSpd] -> Inertia Comp Notch Compensation/2(VehSpd)
  GenFddIcCmd/1(InertiaComp) -> Inertia Comp Notch Compensation/1(InertiaComp)
  If/1 -> InertiaCmpVelCmdDisable/Action
  If/2 -> InertiaCmpVelCmdEnable/Action
  InertiaCmpVelCmdDisable/1(InertiaCmpVelCmd) -> Merge/1
  InertiaCmpVelCmdEnable/1(InertiaCmpVelCmd) -> Merge/2
  Inertia Comp Notch Compensation/1(InertiaCompcompensated) -> InertiaCmpVelCmdEnable/1(InertiaCompcompensated)
  Merge/1 -> LimStat_f32/1
  FltInj_f32/1(Out1) -> InertiaCmpVelCmd/1
  LimStat_f32/1 -> FltInj_f32/1(Signal)
  Constant2/1 -> FltInj_f32/2(Const)
  InertiaCmpVelCmdDi/1 -> If/1
  InertiaCmpDecelGainDi/1 -> ADDCoefCalc/6(InertiaCmpDecelGainDi)

== system SF014A_InertiaCmpVel/InertiaCmpVel/InertiaCmpVelInit1/CopyRight2 ==

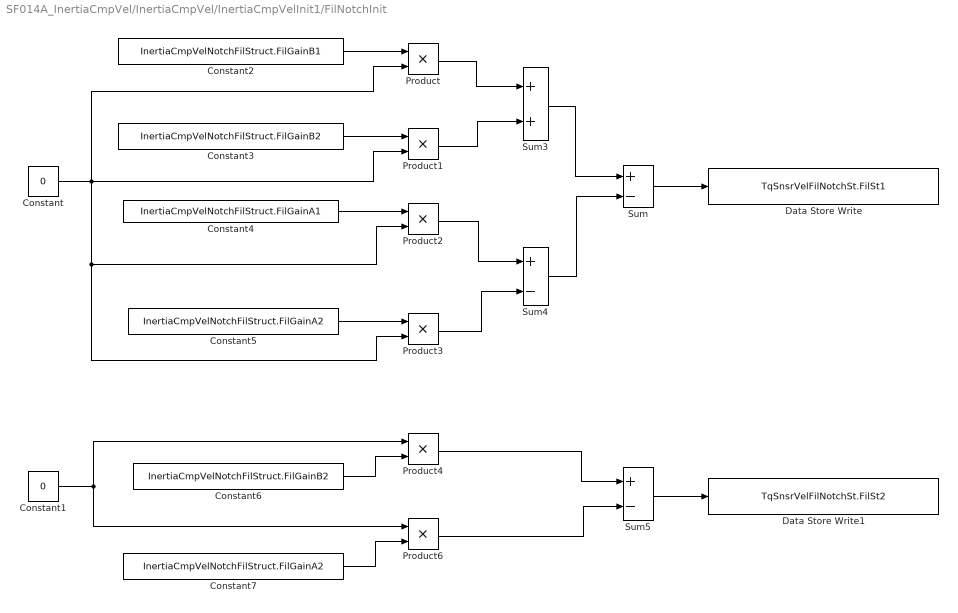
== system SF014A_InertiaCmpVel/InertiaCmpVel/InertiaCmpVelInit1/FilNotchInit ==
  Constant : Constant  Value=0  OutDataTypeStr=single
      settings: AttributesFormatString=%<OutDataTypeStr>
  Constant1 : Constant  Value=0  OutDataTypeStr=single
      settings: AttributesFormatString=%<OutDataTypeStr>
  Constant2 : Constant  Value=InertiaCmpVelNotchFilStruct.FilGainB1
  Constant3 : Constant  Value=InertiaCmpVelNotchFilStruct.FilGainB2
  Constant4 : Constant  Value=InertiaCmpVelNotchFilStruct.FilGainA1
  Constant5 : Constant  Value=InertiaCmpVelNotchFilStruct.FilGainA2
  Constant6 : Constant  Value=InertiaCmpVelNotchFilStruct.FilGainB2
  Constant7 : Constant  Value=InertiaCmpVelNotchFilStruct.FilGainA2
  Data Store Write : DataStoreWrite  DataStoreName=TqSnsrVelFilNotchSt  DataStoreElements=TqSnsrVelFilNotchSt.FilSt1
  Data Store Write1 : DataStoreWrite  DataStoreName=TqSnsrVelFilNotchSt  DataStoreElements=TqSnsrVelFilNotchSt.FilSt2
  Product{,1..4,6} (6 alike) : Product
  Sum : Sum  Inputs=+-
  Sum3 : Sum
  Sum4 : Sum  Inputs=+-
  Sum5 : Sum  Inputs=+-
  wires:
  Product/1 -> Sum3/1
  Product1/1 -> Sum3/2
  Constant/1 -> Product1/2, Product/2, Product2/2, Product3/2
  Product2/1 -> Sum4/1
  Product3/1 -> Sum4/2
  Sum3/1 -> Sum/1
  Sum4/1 -> Sum/2
  Sum/1 -> Data Store Write/1
  Product4/1 -> Sum5/1
  Product6/1 -> Sum5/2
  Constant1/1 -> Product6/1, Product4/1
  Sum5/1 -> Data Store Write1/1
  Constant2/1 -> Product/1
  Constant3/1 -> Product1/1
  Constant4/1 -> Product2/1
  Constant5/1 -> Product3/1
  Constant6/1 -> Product4/2
  Constant7/1 -> Product6/2

== system SF014A_InertiaCmpVel/InertiaCmpVel/InertiaCmpVelInit1/NotchFilterDisable ==
  Action Port : ActionPort  ActionType=then
  Constant: Add to DD (Imported cal?)3 : Constant  Value=false  OutDataTypeStr=boolean
      settings: AttributesFormatString=%<OutDataTypeStr>
  CopyRight2 : Subsystem  Description=|  mask(Copyright Information){none=on}
      | Copyright info block.                                               
      |                                                                     
      | Place copyright information at the top of every subsystem in design.
      mask prompts: none "No parameters"
      mask help: Place copyright information at the top of every subsystem in design.
      mask Display:
      | NxtrConf = 'Nexteer Confidential';
      | 
      | sys = bdroot; %handle for the current model ("system")
      | first = get_param(sys,'Created');
      | first = first(end-3:end);  %year is last four digits
      | 
      | last = get_param(sys,'LastModifiedDate');
      | if isempty(last)
      |     last = datestr(now,'yyyy');
      | else
      |     last = last(end-3:end);
      | end
      | 
      | if strcmp(first,last)
      |     fprintf('%s -- Copyright %s Nexteer',NxtrConf,first)
      | else
      |     fprintf('%s -- %s%s- %s Nexteer',NxtrConf,char(169),first,last)
      | end
  Out1 : Outport
  wires:
  Constant: Add to DD (Imported cal?)3/1 -> Out1/1

== system SF014A_InertiaCmpVel/InertiaCmpVel/InertiaCmpVelInit1/NotchFilterEnable ==
  Action Port : ActionPort  ActionType=else
  Constant: Add to DD (Imported cal?)3 : Constant  Value=true  OutDataTypeStr=boolean
      settings: AttributesFormatString=%<OutDataTypeStr>
  CopyRight2 : Subsystem  Description=|  mask(Copyright Information){none=on}
      | Copyright info block.                                               
      |                                                                     
      | Place copyright information at the top of every subsystem in design.
      mask prompts: none "No parameters"
      mask help: Place copyright information at the top of every subsystem in design.
      mask Display:
      | NxtrConf = 'Nexteer Confidential';
      | 
      | sys = bdroot; %handle for the current model ("system")
      | first = get_param(sys,'Created');
      | first = first(end-3:end);  %year is last four digits
      | 
      | last = get_param(sys,'LastModifiedDate');
      | if isempty(last)
      |     last = datestr(now,'yyyy');
      | else
      |     last = last(end-3:end);
      | end
      | 
      | if strcmp(first,last)
      |     fprintf('%s -- Copyright %s Nexteer',NxtrConf,first)
      | else
      |     fprintf('%s -- %s%s- %s Nexteer',NxtrConf,char(169),first,last)
      | end
  Out1 : Outport
  wires:
  Constant: Add to DD (Imported cal?)3/1 -> Out1/1
